simulink model "data_inspector_Baleka"  (R2025a)
settings: Solver=ode45  StartTime=0.0  StopTime=Sim.time  MaxStep=0.00001  RelTol=1e-12  AbsTol=1e-12
settings Model: Creator=heath  LastModifiedBy=Gavin

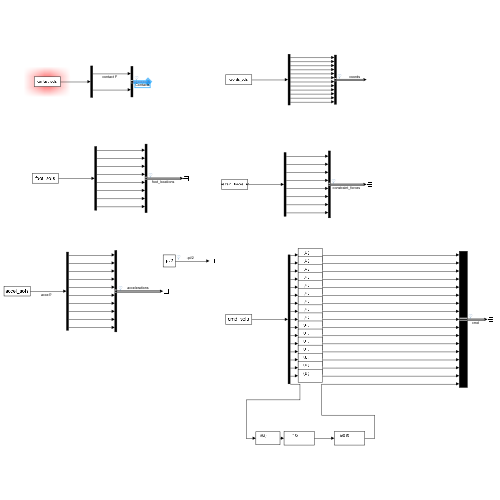
[thumbnail: Simulink's stored preview of the top-level diagram]
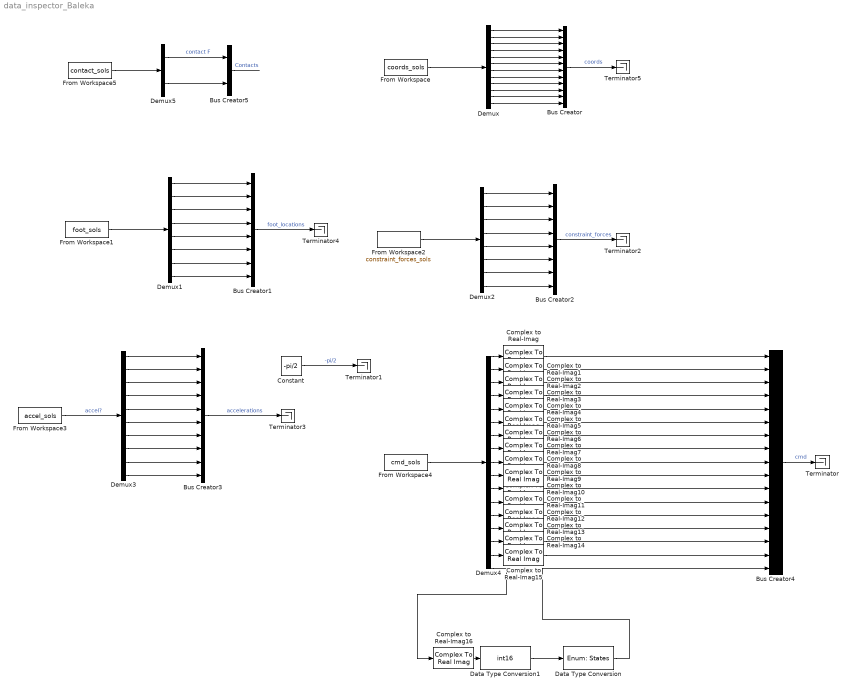
== system data_inspector_Baleka ==
  Bus Creator : BusCreator  Inputs=12  OutDataTypeStr=Bus: Coordinate
      settings: InheritFromInputs=off
  Bus Creator1 : BusCreator  Inputs=8  OutDataTypeStr=Bus: Foot
      settings: InheritFromInputs=off
  Bus Creator2 : BusCreator  Inputs=8  OutDataTypeStr=Bus: ConstraintForces
      settings: InheritFromInputs=off
  Bus Creator3 : BusCreator  Inputs=10  OutDataTypeStr=Bus: Accel
      settings: InheritFromInputs=off
  Bus Creator4 : BusCreator  Inputs=17  OutDataTypeStr=Bus: Cmd
      settings: InheritFromInputs=off
  Bus Creator5 : BusCreator  Inputs=2  OutDataTypeStr=Bus: Contact  NonVirtualBus=on
      settings: InheritFromInputs=off
  Complex to Real-Imag{,1..16} (17 alike) : ComplexToRealImag  Output=Real
  Constant : Constant  Value=-pi/2
  Data Type Conversion : DataTypeConversion  OutDataTypeStr=Enum: States  SaturateOnIntegerOverflow=off  RndMeth=Floor
  Data Type Conversion1 : DataTypeConversion  OutDataTypeStr=int16  SaturateOnIntegerOverflow=off  RndMeth=Floor
  Demux : Demux  Outputs=12
  Demux1 : Demux  Outputs=8
  Demux2 : Demux  Outputs=8
  Demux3 : Demux  Outputs=10
  Demux4 : Demux  Outputs=17
  Demux5 : Demux  Outputs=2
  From Workspace : FromWorkspace  VariableName=coords_sols
  From Workspace1 : FromWorkspace  VariableName=foot_sols
  From Workspace2 : FromWorkspace  VariableName=constraint_forces_sols
  From Workspace3 : FromWorkspace  VariableName=accel_sols
  From Workspace4 : FromWorkspace  VariableName=cmd_sols
  From Workspace5 : FromWorkspace  VariableName=contact_sols
  Terminator{,1..5} (6 alike) : Terminator
  wires:
  From Workspace2/1 -> Demux2/1
  Bus Creator/1 -> Terminator5/1  "coords"
  Demux/8 -> Bus Creator/8
  Demux/7 -> Bus Creator/7
  Demux/6 -> Bus Creator/6
  Demux/5 -> Bus Creator/5
  Demux/4 -> Bus Creator/4
  Demux/3 -> Bus Creator/3
  Demux/2 -> Bus Creator/2
  Demux/1 -> Bus Creator/1
  From Workspace/1 -> Demux/1
  Bus Creator2/1 -> Terminator2/1  "constraint_forces"
  From Workspace4/1 -> Demux4/1
  Bus Creator4/1 -> Terminator/1  "cmd"
  Demux2/4 -> Bus Creator2/4
  Demux2/3 -> Bus Creator2/3
  Demux2/2 -> Bus Creator2/2
  Demux2/1 -> Bus Creator2/1
  Data Type Conversion/1 -> Bus Creator4/17
  Data Type Conversion1/1 -> Data Type Conversion/1
  Demux4/17 -> Complex to Real-Imag16/1
  From Workspace1/1 -> Demux1/1
  Demux1/4 -> Bus Creator1/4
  Demux1/2 -> Bus Creator1/2
  Demux1/1 -> Bus Creator1/1
  Bus Creator1/1 -> Terminator4/1  "foot_locations"
  Demux1/3 -> Bus Creator1/3
  Constant/1 -> Terminator1/1  "-pi/2"
  Bus Creator3/1 -> Terminator3/1  "accelerations"
  Demux3/4 -> Bus Creator3/4
  Demux3/1 -> Bus Creator3/1
  From Workspace3/1 -> Demux3/1  "accel?"
  Demux3/3 -> Bus Creator3/3
  Demux3/2 -> Bus Creator3/2
  Demux3/5 -> Bus Creator3/5
  Demux3/6 -> Bus Creator3/6
  Demux1/5 -> Bus Creator1/5
  Demux1/6 -> Bus Creator1/6
  Demux1/7 -> Bus Creator1/7
  Demux1/8 -> Bus Creator1/8
  Demux3/7 -> Bus Creator3/7
  Demux3/8 -> Bus Creator3/8
  Demux3/9 -> Bus Creator3/9
  Demux3/10 -> Bus Creator3/10
  Demux/9 -> Bus Creator/9
  Demux/10 -> Bus Creator/10
  Demux/11 -> Bus Creator/11
  Demux/12 -> Bus Creator/12
  Demux2/8 -> Bus Creator2/8
  Demux2/7 -> Bus Creator2/7
  Demux2/6 -> Bus Creator2/6
  Demux2/5 -> Bus Creator2/5
  Demux4/1 -> Complex to Real-Imag/1
  Demux4/2 -> Complex to Real-Imag1/1
  Complex to Real-Imag1/1 -> Bus Creator4/2
  Complex to Real-Imag/1 -> Bus Creator4/1
  Complex to Real-Imag2/1 -> Bus Creator4/3
  Demux4/3 -> Complex to Real-Imag2/1
  Demux4/4 -> Complex to Real-Imag3/1
  Complex to Real-Imag3/1 -> Bus Creator4/4
  Demux4/5 -> Complex to Real-Imag4/1
  Complex to Real-Imag4/1 -> Bus Creator4/5
  Demux4/6 -> Complex to Real-Imag5/1
  Complex to Real-Imag5/1 -> Bus Creator4/6
  Demux4/7 -> Complex to Real-Imag6/1
  Complex to Real-Imag6/1 -> Bus Creator4/7
  Demux4/8 -> Complex to Real-Imag7/1
  Complex to Real-Imag7/1 -> Bus Creator4/8
  Demux4/9 -> Complex to Real-Imag8/1
  Complex to Real-Imag8/1 -> Bus Creator4/9
  Demux4/10 -> Complex to Real-Imag9/1
  Complex to Real-Imag9/1 -> Bus Creator4/10
  Demux4/11 -> Complex to Real-Imag10/1
  Complex to Real-Imag10/1 -> Bus Creator4/11
  Demux4/12 -> Complex to Real-Imag11/1
  Complex to Real-Imag11/1 -> Bus Creator4/12
  Demux4/13 -> Complex to Real-Imag12/1
  Complex to Real-Imag12/1 -> Bus Creator4/13
  Demux4/14 -> Complex to Real-Imag13/1
  Complex to Real-Imag13/1 -> Bus Creator4/14
  Demux4/15 -> Complex to Real-Imag14/1
  Complex to Real-Imag14/1 -> Bus Creator4/15
  Demux4/16 -> Complex to Real-Imag15/1
  Complex to Real-Imag15/1 -> Bus Creator4/16
  Complex to Real-Imag16/1 -> Data Type Conversion1/1
  From Workspace5/1 -> Demux5/1
  Demux5/1 -> Bus Creator5/1  "contact F"
  Demux5/2 -> Bus Creator5/2
  Bus Creator5/1 -> ?  "Contacts"
